simulink model "MEKFsim_v2"  (R2020b)
settings: Solver=FixedStepAuto  StartTime=0.0  StopTime=tsimulation  FixedStep=delta_t  RelTol=1e-3
values from neighbouring files (symbols this model uses):
  b_offset = sat.sensors.gyro_bias    [MEKF_Monte_Carlo_simulation.m]    (also in UKF_Monte_Carlo_simulation.m; main_SDA.m; main_SDA_v2.m)
  b_offset2 = -1e-2    (= -0.01)    [MEKF_Monte_Carlo_simulation.m]    (also in UKF_Monte_Carlo_simulation.m; main_SDA.m = 0; main_SDA_v2.m = 0)
  date_IGRF = [date.year,date.month,date.day]    [MEKF_Monte_Carlo_simulation.m]    (also in UKF_Monte_Carlo_simulation.m; main_SDA.m; main_SDA_v2.m)
  m = 12    [MEKF_Monte_Carlo_simulation.m]    (also in UKF_Monte_Carlo_simulation.m; main_SDA.m; main_SDA_v2.m)
  MODE = 2    [MEKF_Monte_Carlo_simulation.m]    (also in UKF_Monte_Carlo_simulation.m; main_SDA.m; main_SDA_v2.m)
  nmax_KF = 2    [MEKF_Monte_Carlo_simulation.m]    (also in UKF_Monte_Carlo_simulation.m; main_SDA.m; main_SDA_v2.m)
  PSDbias = sat.sensors.gyro_bias^2*Ts    [MEKF_Monte_Carlo_simulation.m]    (also in UKF_Monte_Carlo_simulation.m; main_SDA.m; main_SDA_v2.m)
  PSDcss = sat.sensors.sun_coarse_sigma^2*Tss    [MEKF_Monte_Carlo_simulation.m]    (also in UKF_Monte_Carlo_simulation.m; main_SDA.m; main_SDA_v2.m)
  PSDfss = sat.sensors.sun_sigma^2*Tss    [MEKF_Monte_Carlo_simulation.m]    (also in UKF_Monte_Carlo_simulation.m; main_SDA.m; main_SDA_v2.m)
  PSDgyro = sat.sensors.gyro_sigma^2*Ts    [MEKF_Monte_Carlo_simulation.m]    (also in UKF_Monte_Carlo_simulation.m; main_SDA.m; main_SDA_v2.m)
  PSDmtm = sat.sensors.mag_sigma^2*Tss    [MEKF_Monte_Carlo_simulation.m]    (also in UKF_Monte_Carlo_simulation.m; main_SDA.m; main_SDA_v2.m)
  Ts = 1    [MEKF_Monte_Carlo_simulation.m]    (also in UKF_Monte_Carlo_simulation.m; main_SDA.m = 0.5; main_SDA_v2.m = 0.5)
  Tss = 1    [MEKF_Monte_Carlo_simulation.m]    (also in UKF_Monte_Carlo_simulation.m; main_SDA.m = 0.5; main_SDA_v2.m = 0.5)
  Use_IGRF = 0    [MEKF_Monte_Carlo_simulation.m]    (also in UKF_Monte_Carlo_simulation.m; main_SDA.m; main_SDA_v2.m)
  Use_IGRF_KF = 0    [MEKF_Monte_Carlo_simulation.m]    (also in UKF_Monte_Carlo_simulation.m; main_SDA.m; main_SDA_v2.m)
undefined symbols (not defined in the file or in its folder): date, deg, DipoleMod, km, orbit, rad, s
libraries: aerolibconvert2 x14, aerolibutil x14, sharedtransform x9, dspmathops x8, vrlib x7, simulink x6, aerolibobsolete x2, aerolibcelestial x2, aerolibgravity2 x1, sharedutil x1, DipoleModel x1
(part 1 of 2)
settings Model: Creator=Ricardo  LastModifiedBy=colpari

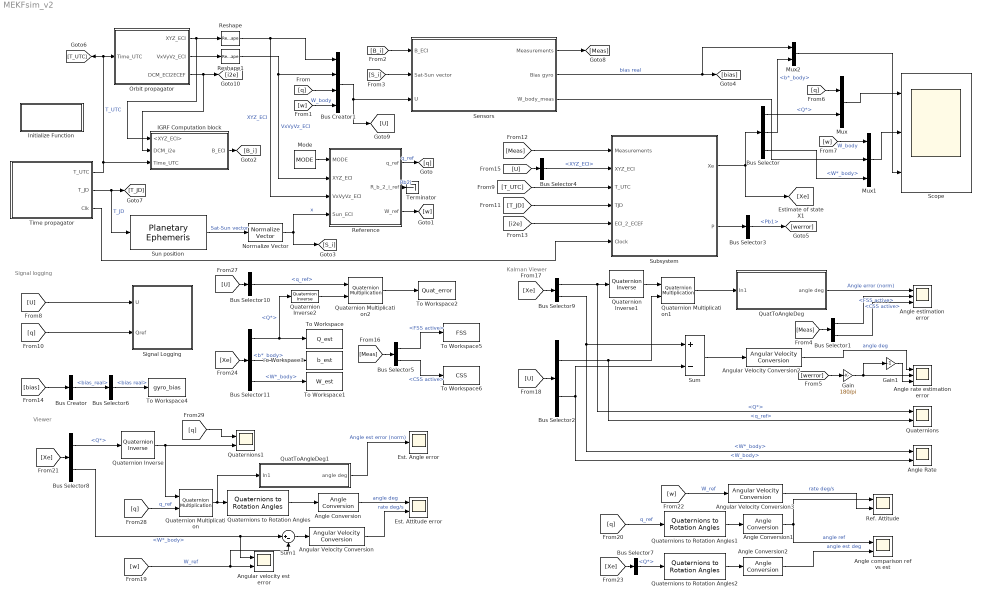
== system MEKFsim_v2 ==
  note: Signal logging
  note: Kalman Viewer
  note: Viewer
  Angle comparison ref vs est : Scope  NumInputPorts=2
  Angle Conversion : aerolibconvert2/Angle Conversion  IU=rad  OU=deg
  Angle Conversion1 : aerolibconvert2/Angle Conversion  IU=rad  OU=deg
  Angle Conversion2 : aerolibconvert2/Angle Conversion  IU=rad  OU=deg
  Angle Rate : Scope  NumInputPorts=2
  Angle estimation error : Scope  NumInputPorts=3
  Angle rate estimation error : Scope  NumInputPorts=3
  Angular Velocity Conversion : aerolibconvert2/Angular Velocity Conversion  IU=rad/s  OU=deg/s
  Angular Velocity Conversion2 : aerolibconvert2/Angular Velocity Conversion  IU=rad/s  OU=deg/s
  Angular Velocity Conversion3 : aerolibconvert2/Angular Velocity Conversion  IU=rad/s  OU=deg/s
  Angular velocity est error : Scope  NumInputPorts=2
  Bus Creator : BusCreator  Inputs=1
  Bus Creator1 : BusCreator  Inputs=4
  Bus Selector : BusSelector  OutputSignals=Q*,b*_body,W*_body
  Bus Selector1 : BusSelector  OutputSignals=FSS active,CSS active
  Bus Selector10 : BusSelector  OutputSignals=q_ref
  Bus Selector11 : BusSelector  OutputSignals=Q*,b*_body,W*_body
  Bus Selector2 : BusSelector  OutputSignals=q_ref,W_body
  Bus Selector3 : BusSelector  OutputSignals=Pb1
  Bus Selector4 : BusSelector  OutputSignals=XYZ_ECI
  Bus Selector5 : BusSelector  OutputSignals=FSS active,CSS active
  Bus Selector6 : BusSelector  OutputSignals=bias real
  Bus Selector7 : BusSelector  OutputSignals=Q*
  Bus Selector8 : BusSelector  OutputSignals=Q*,W*_body
  Bus Selector9 : BusSelector  OutputSignals=Q*,W*_body
  Est. Angle error : Scope
  Est. Attitude error : Scope  NumInputPorts=2
  Gain : Gain  Gain=180/pi
  Gain1 : Gain  Gain=-1
  IGRF Computation block : Subsystem
  Initialize Function : Subsystem  TreatAsAtomicUnit=on
  Mode : Constant  Value=MODE  OutDataTypeStr=int8
  Mux : Mux  Inputs=2
  Mux1 : Mux  Inputs=3
  Mux2 : Mux  Inputs=2
  Normalize Vector : vrlib/Utilities/Normalize Vector  maxzero=0
  Orbit propagator : Subsystem
  QuatToAngleDeg : Subsystem
  QuatToAngleDeg1 : Subsystem
  Quaternion Inverse : aerolibutil/Quaternion Inverse
  Quaternion Inverse1 : aerolibutil/Quaternion Inverse
  Quaternion Inverse2 : aerolibutil/Quaternion Inverse
  Quaternion Multiplication : aerolibutil/Quaternion Multiplication
  Quaternion Multiplication1 : aerolibutil/Quaternion Multiplication
  Quaternion Multiplication2 : aerolibutil/Quaternion Multiplication
  Quaternions : Scope  NumInputPorts=2
  Quaternions to Rotation Angles : sharedtransform/Quaternions to Rotation Angles  rotationOrder=ZYX  aMode=aMode
      settings: SourceProductBaseCode=AE,PW,MT,UV,VE,VP
  Quaternions to Rotation Angles1 : sharedtransform/Quaternions to Rotation Angles  rotationOrder=ZYX  aMode=aMode
      settings: SourceProductBaseCode=AE,PW,MT,UV,VE,VP
  Quaternions to Rotation Angles2 : sharedtransform/Quaternions to Rotation Angles  rotationOrder=ZYX  aMode=aMode
      settings: SourceProductBaseCode=AE,PW,MT,UV,VE,VP
  Quaternions1 : Scope  NumInputPorts=2
  Ref. Attitude : Scope  NumInputPorts=2
  Reference : Subsystem  TreatAsAtomicUnit=on
  Reshape : Reshape
  Reshape1 : Reshape
  Scope : Scope  NumInputPorts=3
  Sensors : Subsystem
  Signal Logging : Subsystem
  Subsystem : Subsystem
  Sum : Sum  Inputs=+-
  Sum1 : Sum  Inputs=|+-
  Sun position : aerolibcelestial/Planetary Ephemeris  kmflag=km,km/s  epochflag=Julian date  de=DE405  nCenter=Earth  nTarget=Sun  errorflag=Error  velflag=off
      settings: SourceProductBaseCode=AE
  Terminator : Terminator
  Time propagator : Subsystem
  To Workspace : ToWorkspace  VariableName=Q_est  SaveFormat=Timeseries  SampleTime=-1
  To Workspace1 : ToWorkspace  VariableName=W_est  SaveFormat=Timeseries  SampleTime=-1
  To Workspace2 : ToWorkspace  VariableName=Quat_error  SaveFormat=Timeseries  SampleTime=-1
  To Workspace3 : ToWorkspace  VariableName=b_est  SaveFormat=Timeseries  SampleTime=-1
  To Workspace4 : ToWorkspace  VariableName=gyro_bias  SaveFormat=Timeseries  SampleTime=-1
      settings: Save2DSignal=2-D array (concatenate along first dimension)
  To Workspace5 : ToWorkspace  VariableName=FSS  SaveFormat=Timeseries  SampleTime=-1
  To Workspace6 : ToWorkspace  VariableName=CSS  SaveFormat=Timeseries  SampleTime=-1
  wires:
  Orbit propagator/2(VxVyVz_ECI) -> Reshape1/1
  Orbit propagator/1(XYZ_ECI) -> IGRF Computation block/1(<XYZ_ECI>), Reshape/1
  Normalize Vector/1 -> Reference/4(Sun_ECI), [S_i]  "x"
  Sun position/1 -> Normalize Vector/1  "Sat-Sun vector"
  Time propagator/1(T_UTC) -> IGRF Computation block/3("Time_UTC "), [T_UTC], Orbit propagator/1("Time_UTC ")  "T_UTC"
  Time propagator/2(T_JD) -> Sun position/1, [T_JD]  "T_JD"
  Orbit propagator/3(DCM_ECI2ECEF) -> IGRF Computation block/2("DCM_i2e "), [i2e]
  IGRF Computation block/1(B_ECI) -> [B_i]
  [q] -> Bus Creator1/3
  [w] -> Bus Creator1/4  "W_body"
  Bus Creator1/1 -> [U], Sensors/3(U)
  [B_i] -> Sensors/1(B_ECI)
  [S_i] -> Sensors/2(Sat-Sun vector)
  [q] -> Mux/1
  Bus Selector/1 -> Mux/2  "<Q*>"
  Bus Selector/3 -> Mux1/3  "<W*_body>"
  [w] -> Mux1/1  "W_body"
  Sensors/3(W_body_meas) -> Mux1/2
  Mux/1 -> Scope/1
  Mux1/1 -> Scope/2
  Bus Selector11/1 -> Quaternion Inverse2/1, To Workspace/1  "<Q*>"
  Bus Selector10/1 -> Quaternion Multiplication2/1  "<q_ref>"
  [q] -> Signal Logging/2(Qref)
  Quaternion Inverse2/1 -> Quaternion Multiplication2/2
  Quaternion Multiplication2/1 -> To Workspace2/1
  [U] -> Bus Selector10/1
  [Xe] -> Bus Selector11/1
  [U] -> Signal Logging/1(U)
  Bus Selector11/3 -> To Workspace1/1  "<W*_body>"
  Quaternion Multiplication1/1 -> QuatToAngleDeg/1(In1)
  Bus Selector1/2 -> Angle estimation error/3  "<CSS active>"
  QuatToAngleDeg/1(angle deg) -> Angle estimation error/1  "Angle error (norm)"
  Angular Velocity Conversion2/1 -> Angle rate estimation error/1  "angle deg"
  Bus Selector2/1 -> Quaternions/2, Quaternion Multiplication1/2  "<q_ref>"
  Bus Selector1/1 -> Angle estimation error/2  "<FSS active>"
  Bus Selector2/2 -> Sum/2, Angle Rate/2  "<W_body>"
  Sum/1 -> Angular Velocity Conversion2/1
  [Xe] -> Bus Selector9/1
  Bus Selector9/1 -> Quaternions/1, Quaternion Inverse1/1  "<Q*>"
  Bus Selector9/2 -> Angle Rate/1, Sum/1  "<W*_body>"
  Quaternion Inverse1/1 -> Quaternion Multiplication1/1
  [U] -> Bus Selector2/1
  [T_UTC] -> Subsystem/3(T_UTC)
  [T_JD] -> Subsystem/4(TJD)
  Bus Selector4/1 -> Subsystem/2(XYZ_ECI)  "<XYZ_ECI>"
  [U] -> Bus Selector4/1
  Subsystem/1(Xe) -> [Xe], Bus Selector/1
  Subsystem/2(P) -> Bus Selector3/1
  Gain1/1 -> Angle rate estimation error/3
  Bus Selector3/1 -> [werror]  "<Pb1>"
  [werror] -> Gain/1
  Gain/1 -> Gain1/1, Angle rate estimation error/2
  Reshape1/1 -> Reference/2(XYZ_ECI), Bus Creator1/2  "VxVyVz_ECI"
  Reshape/1 -> Reference/3(VxVyVz_ECI), Bus Creator1/1  "XYZ_ECI"
  [i2e] -> Subsystem/5(ECI_2_ECEF)
  Time propagator/3(Clk) -> Subsystem/6(Clock)
  Sensors/2(Bias gyro) -> [bias], Mux2/1  "bias real"
  Bus Selector/2 -> Mux2/2  "<b*_body>"
  Mux2/1 -> Scope/3
  Sensors/1(Measurements) -> [Meas]
  [Meas] -> Subsystem/1(Measurements)
  [Meas] -> Bus Selector1/1
  Bus Selector11/2 -> To Workspace3/1  "<b*_body>"
  [bias] -> Bus Creator/1
  Bus Selector5/1 -> To Workspace5/1  "<FSS active>"
  [Meas] -> Bus Selector5/1
  Bus Selector5/2 -> To Workspace6/1  "<CSS active>"
  Bus Creator/1 -> Bus Selector6/1  "<bias_real>"
  Bus Selector6/1 -> To Workspace4/1  "<bias real>"
  Reference/2(R_b_2_i_ref) -> Terminator/1  "Rb2i"
  Reference/1(q_ref) -> [q]  "q_ref"
  Reference/3(W_ref) -> [w]
  Mode/1 -> Reference/1(MODE)
  Bus Selector8/1 -> Quaternion Inverse/1  "<Q*>"
  [q] -> Quaternion Multiplication/2  "q_ref"
  Quaternions to Rotation Angles/1 -> Angle Conversion/1
  [w] -> Sum1/2, Angular velocity est error/2  "W_ref"
  Quaternion Inverse/1 -> Quaternion Multiplication/1, Quaternions1/2
  [Xe] -> Bus Selector8/1
  Angle Conversion/1 -> Est. Attitude error/1  "angle deg"
  QuatToAngleDeg1/1(angle deg) -> Est. Angle error/1  "Angle est error (norm)"
  Quaternion Multiplication/1 -> QuatToAngleDeg1/1(In1), Quaternions to Rotation Angles/1
  Sum1/1 -> Angular Velocity Conversion/1
  Angular Velocity Conversion/1 -> Est. Attitude error/2  "rate deg/s"
  [q] -> Quaternions1/1
  Bus Selector8/2 -> Sum1/1, Angular velocity est error/1  "<W*_body>"
  [w] -> Angular Velocity Conversion3/1  "W_ref"
  [Xe] -> Bus Selector7/1
  Angular Velocity Conversion3/1 -> Ref. Attitude/2  "rate deg/s"
  Angle Conversion2/1 -> Angle comparison ref vs est/2  "angle est deg"
  Bus Selector7/1 -> Quaternions to Rotation Angles2/1  "<Q*>"
  Quaternions to Rotation Angles1/1 -> Angle Conversion1/1
  Angle Conversion1/1 -> Ref. Attitude/1, Angle comparison ref vs est/1  "angle ref"
  Quaternions to Rotation Angles2/1 -> Angle Conversion2/1
  [q] -> Quaternions to Rotation Angles1/1  "q_ref"

== system MEKFsim_v2/IGRF Computation block ==
  <XYZ_ECI> : Inport
  "DCM_i2e " : Inport  Port=2
  "Time_UTC " : Inport  Port=3
  Bus Creator : BusCreator  Inputs=5
  Demux : Demux  Outputs=2
  ECI To LLA : MATLAB Function  TreatAsAtomicUnit=on
  Obtain B_ECI : Subsystem
  Product : Product  Multiplication=Matrix(*)
  Reshape : Reshape  OutputDimensionality=Row vector (2-D)
  Terminator : Terminator
  B_ECI : Outport  VectorParamsAs1DForOutWhenUnconnected=off
  wires:
  ECI To LLA/3(long) -> Bus Creator/3
  ECI To LLA/2(lat) -> Bus Creator/2
  ECI To LLA/1(h) -> Bus Creator/1
  Demux/1 -> Bus Creator/4  "time_UTC"
  Demux/2 -> Terminator/1
  "DCM_i2e "/1 -> Product/2, Bus Creator/5  "DCM_i2e"
  Reshape/1 -> Product/1
  Product/1 -> ECI To LLA/1(X_ECEF)
  Bus Creator/1 -> Obtain B_ECI/1(In1)
  Obtain B_ECI/1(Out1) -> B_ECI/1
  "Time_UTC "/1 -> Demux/1
  <XYZ_ECI>/1 -> Reshape/1

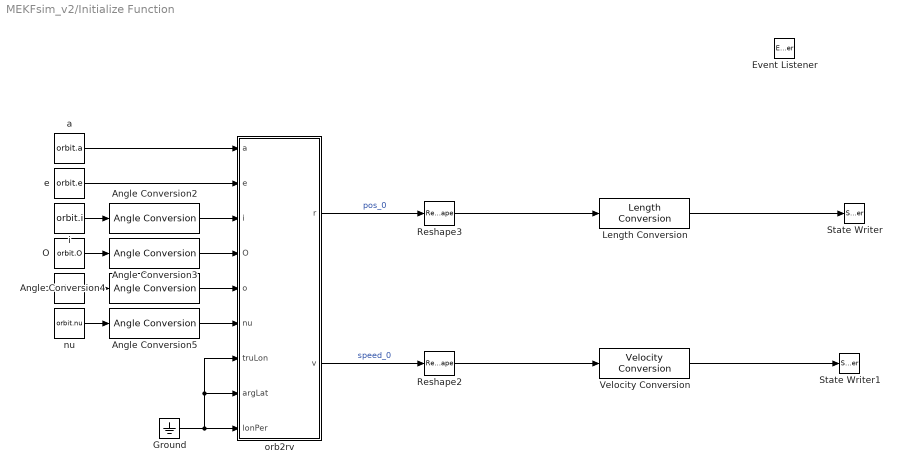
== system MEKFsim_v2/Initialize Function ==
  Angle Conversion{2..5} (4 alike) : aerolibconvert2/Angle Conversion  IU=deg  OU=rad
  Event Listener : EventListener  DisableCoverage=on  EventName=reset
  Ground : Ground
  Length Conversion : aerolibconvert2/Length Conversion  IU=km  OU=m
  O : Constant  Value=orbit.O
  Reshape2 : Reshape  OutputDimensionality=Column vector (2-D)
  Reshape3 : Reshape  OutputDimensionality=Column vector (2-D)
  State Writer : StateWriter  StateOwnerBlock=../../Orbit propagator/Integrator_pos
  State Writer1 : StateWriter  StateOwnerBlock=../../Orbit propagator/Integrator_speed
  Velocity Conversion : aerolibconvert2/Velocity Conversion  IU=km/s  OU=m/s
  a : Constant  Value=orbit.a
  e : Constant  Value=orbit.e
  i : Constant  Value=orbit.i
  nu : Constant  Value=orbit.nu
  o : Constant  Value=orbit.o
  orb2rv : MATLAB Function  TreatAsAtomicUnit=on
  wires:
  Angle Conversion2/1 -> orb2rv/3(i)
  Length Conversion/1 -> State Writer/1
  Angle Conversion4/1 -> orb2rv/5(o)
  nu/1 -> Angle Conversion5/1
  Angle Conversion3/1 -> orb2rv/4(O)
  e/1 -> orb2rv/2(e)
  Reshape3/1 -> Length Conversion/1
  O/1 -> Angle Conversion3/1
  a/1 -> orb2rv/1(a)
  i/1 -> Angle Conversion2/1
  orb2rv/1(r) -> Reshape3/1  "pos_0"
  o/1 -> Angle Conversion4/1
  Angle Conversion5/1 -> orb2rv/6(nu)
  Velocity Conversion/1 -> State Writer1/1
  Reshape2/1 -> Velocity Conversion/1
  orb2rv/2(v) -> Reshape2/1  "speed_0"
  Ground/1 -> orb2rv/8(argLat), orb2rv/7(truLon), orb2rv/9(lonPer)

== system MEKFsim_v2/Orbit propagator ==
  "Time_UTC " : Inport
  1/m : Gain  Gain=1/m
  Integrator_pos : Integrator
  Integrator_speed : Integrator
  Reshape : Reshape  OutputDimensionality=Column vector (2-D)
  Reshape2 : Reshape  OutputDimensionality=Column vector (2-D)
  Spherical Harmonic Gravity : Subsystem  TreatAsAtomicUnit=on  SystemSampleTime=1
  m : Gain  Gain=m
  XYZ_ECI : Outport  VectorParamsAs1DForOutWhenUnconnected=off
  VxVyVz_ECI : Outport  Port=2
  DCM_ECI2ECEF : Outport  Port=3
  wires:
  Integrator_pos/1 -> Reshape2/1, XYZ_ECI/1  "XYZ_ECI"
  Integrator_speed/1 -> VxVyVz_ECI/1, Integrator_pos/1  "VxVyVz_ECI"
  1/m/1 -> Integrator_speed/1  "AxAyAz_ECI"
  Reshape/1 -> 1/m/1
  m/1 -> Reshape/1  "Force_ECI"
  Spherical Harmonic Gravity/1(g_ECI (m/s²)) -> m/1
  "Time_UTC "/1 -> Spherical Harmonic Gravity/2(Time_UTC)
  Reshape2/1 -> Spherical Harmonic Gravity/1(XYZ_ECI)
  Spherical Harmonic Gravity/2(DCM_ECI2ECEF) -> DCM_ECI2ECEF/1

== system MEKFsim_v2/QuatToAngleDeg ==
  In1 : Inport
  Abs : Abs
  Abs1 : Abs
  Acos : Trigonometry  Operator=acos
  Angle Conversion1 : aerolibconvert2/Angle Conversion  IU=rad  OU=deg
  Demux1 : Demux
  Gain : Gain  Gain=2
  Scope : Scope
  Terminator1 : Terminator
  Terminator2 : Terminator
  Terminator3 : Terminator
  angle deg : Outport  VectorParamsAs1DForOutWhenUnconnected=off
  wires:
  Acos/1 -> Gain/1
  Demux1/4 -> Terminator1/1
  In1/1 -> Demux1/1
  Angle Conversion1/1 -> Abs/1  "angle deg"
  Demux1/2 -> Terminator2/1
  Demux1/3 -> Terminator3/1
  Abs/1 -> angle deg/1
  Demux1/1 -> Abs1/1, Scope/1
  Gain/1 -> Angle Conversion1/1
  Abs1/1 -> Acos/1

== system MEKFsim_v2/QuatToAngleDeg1 ==
  In1 : Inport
  Abs : Abs
  Angle Conversion1 : aerolibconvert2/Angle Conversion  IU=rad  OU=deg
  Demux1 : Demux
  Quaternion to axis and angle conversion : MATLABFcn  MATLABFcn=quat2axisangle
  Terminator1 : Terminator
  Terminator2 : Terminator
  Terminator3 : Terminator
  angle deg : Outport  VectorParamsAs1DForOutWhenUnconnected=off
  wires:
  Demux1/2 -> Terminator2/1
  Demux1/4 -> Angle Conversion1/1
  In1/1 -> Quaternion to axis and angle conversion/1
  Demux1/1 -> Terminator1/1
  Demux1/3 -> Terminator3/1
  Quaternion to axis and angle conversion/1 -> Demux1/1
  Abs/1 -> angle deg/1
  Angle Conversion1/1 -> Abs/1  "angle deg"

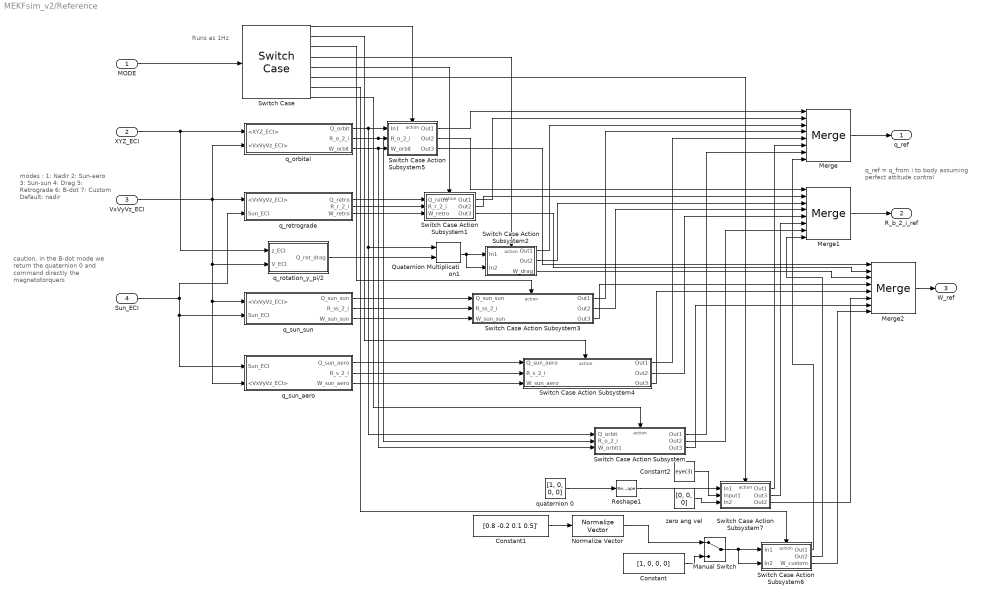
== system MEKFsim_v2/Reference ==
  note: caution, in the B-dot mode we return the quaternion 0 and command directly the magnetotorquers
  note: modes :
      | 1: Nadir
      | 2: Sun-aero
      | 3: Sun-sun
      | 4: Drag
      | 5: Retrograde
      | 6: B-dot
      | 7: Custom
      | Default: nadir
  note: Runs as 1Hz
  note: q_ref  = q_from i to body
      | assuming perfect attitude control
  MODE : Inport  OutMin=1  OutMax=100  OutDataTypeStr=int8
  XYZ_ECI : Inport  Port=2
  VxVyVz_ECI : Inport  Port=3
  Sun_ECI : Inport  Port=4
  Constant : Constant  Value=[1, 0, 0, 0]
  Constant1 : Constant  Value=[0.8 -0.2 0.1 0.5]'
  Constant2 : Constant  Value=eye(3)
  Manual Switch : ManualSwitch
  Merge : Merge  Inputs=8
  Merge1 : Merge  Inputs=8
  Merge2 : Merge  Inputs=8
  Normalize Vector : vrlib/Utilities/Normalize Vector  maxzero=0
  Quaternion Multiplication1 : aerolibutil/Quaternion Multiplication
  Reshape1 : Reshape  OutputDimensionality=Column vector (2-D)
  Switch Case : SwitchCase  CaseConditions={1, 2, 3, 4, 5, 6, 7}
  Switch Case Action Subsystem : Subsystem  TreatAsAtomicUnit=on
  Switch Case Action Subsystem1 : Subsystem  TreatAsAtomicUnit=on
  Switch Case Action Subsystem2 : Subsystem  TreatAsAtomicUnit=on
  Switch Case Action Subsystem3 : Subsystem  TreatAsAtomicUnit=on
  Switch Case Action Subsystem4 : Subsystem  TreatAsAtomicUnit=on
  Switch Case Action Subsystem5 : Subsystem  TreatAsAtomicUnit=on
  Switch Case Action Subsystem6 : Subsystem  TreatAsAtomicUnit=on
  Switch Case Action Subsystem7 : Subsystem  TreatAsAtomicUnit=on
  q_orbital : Subsystem
  q_retrograde : Subsystem
  q_rotation_y_pi/2 : Subsystem
  q_sun_aero : Subsystem
  q_sun_sun : Subsystem
  quaternion 0 : Constant  Value=[1, 0, 0, 0]
  zero ang vel : Constant  Value=[0, 0, 0]
  q_ref : Outport  VectorParamsAs1DForOutWhenUnconnected=off
  R_b_2_i_ref : Outport  Port=2
  W_ref : Outport  Port=3
  wires:
  q_sun_sun/1(Q_sun_sun) -> Switch Case Action Subsystem3/1(Q_sun_sun)
  Sun_ECI/1 -> q_retrograde/2(Sun_ECI), q_sun_aero/1(Sun_ECI), q_sun_sun/2(Sun_ECI)
  MODE/1 -> Switch Case/1
  q_rotation_y_pi/2/1(Q_rot_drag) -> Quaternion Multiplication1/2
  Switch Case/3 -> Switch Case Action Subsystem3/Action
  q_sun_aero/1(Q_sun_aero) -> Switch Case Action Subsystem4/1(Q_sun_aero)
  Merge/1 -> q_ref/1
  XYZ_ECI/1 -> q_orbital/1(<XYZ_ECI>), q_rotation_y_pi/2/1(z_ECI)
  Switch Case/5 -> Switch Case Action Subsystem1/Action
  Switch Case/4 -> Switch Case Action Subsystem2/Action
  quaternion 0/1 -> Reshape1/1
  VxVyVz_ECI/1 -> q_orbital/2(<VxVyVz_ECI>), q_retrograde/1(<VxVyVz_ECI>), q_sun_aero/2(<VxVyVz_ECI>), q_sun_sun/1(<VxVyVz_ECI>), q_rotation_y_pi/2/2(V_ECI)
  Switch Case/2 -> Switch Case Action Subsystem4/Action
  Quaternion Multiplication1/1 -> Switch Case Action Subsystem2/2(In2), Switch Case Action Subsystem2/1(In1)
  q_orbital/1(Q_orbit) -> Quaternion Multiplication1/1, Switch Case Action Subsystem/1(Q_orbit), Switch Case Action Subsystem5/1(In1)
  Switch Case/6 -> Switch Case Action Subsystem7/Action
  q_retrograde/1(Q_retro) -> Switch Case Action Subsystem1/1(Q_retro)
  Reshape1/1 -> Switch Case Action Subsystem7/1(In1)
  Merge1/1 -> R_b_2_i_ref/1
  Switch Case Action Subsystem5/1(Out1) -> Merge/1
  Switch Case Action Subsystem5/2(Out2) -> Merge1/1
  Switch Case Action Subsystem1/1(Out1) -> Merge/2
  Switch Case Action Subsystem1/2(Out2) -> Merge1/2
  Switch Case Action Subsystem2/1(Out1) -> Merge/3
  Switch Case Action Subsystem2/2(Out2) -> Merge1/3
  Switch Case Action Subsystem3/1(Out1) -> Merge/4
  Switch Case Action Subsystem3/2(Out2) -> Merge1/4
  Switch Case Action Subsystem4/1(Out1) -> Merge/5
  Switch Case Action Subsystem4/2(Out2) -> Merge1/5
  Switch Case Action Subsystem/1(Out1) -> Merge/7
  Switch Case Action Subsystem/2(Out2) -> Merge1/7
  Switch Case Action Subsystem7/1(Out1) -> Merge/6
  Switch Case Action Subsystem7/2(Out3) -> Merge1/6
  Switch Case/1 -> Switch Case Action Subsystem5/Action
  Switch Case/8 -> Switch Case Action Subsystem/Action
  Switch Case/7 -> Switch Case Action Subsystem6/Action
  Constant/1 -> Manual Switch/2
  Switch Case Action Subsystem6/1(Out1) -> Merge/8
  Switch Case Action Subsystem6/2(Out2) -> Merge1/8
  Constant1/1 -> Normalize Vector/1
  Normalize Vector/1 -> Manual Switch/1
  Manual Switch/1 -> Switch Case Action Subsystem6/2(In2), Switch Case Action Subsystem6/1(In1)
  q_orbital/2(R_o_2_i) -> Switch Case Action Subsystem/2(R_o_2_i), Switch Case Action Subsystem5/2(R_o_2_i)
  q_sun_aero/2(R_s_2_i) -> Switch Case Action Subsystem4/2(R_s_2_i)
  q_sun_sun/2(R_ss_2_i) -> Switch Case Action Subsystem3/2(R_ss_2_i)
  q_retrograde/2(R_r_2_i) -> Switch Case Action Subsystem1/2(R_r_2_i)
  Constant2/1 -> Switch Case Action Subsystem7/2(Input1)
  q_orbital/3(W_orbit) -> Switch Case Action Subsystem/3(W_orbit1), Switch Case Action Subsystem5/3(W_orbit)
  q_retrograde/3(W_retro) -> Switch Case Action Subsystem1/3(W_retro)
  q_sun_aero/3(W_sun_aero) -> Switch Case Action Subsystem4/3(W_sun_aero)
  q_sun_sun/3(W_sun_sun) -> Switch Case Action Subsystem3/3(W_sun_sun)
  Merge2/1 -> W_ref/1
  Switch Case Action Subsystem5/3(Out3) -> Merge2/1
  Switch Case Action Subsystem4/3(Out3) -> Merge2/5
  Switch Case Action Subsystem3/3(Out3) -> Merge2/4
  Switch Case Action Subsystem2/3(W_drag) -> Merge2/3
  Switch Case Action Subsystem1/3(Out3) -> Merge2/2
  zero ang vel/1 -> Switch Case Action Subsystem7/3(In2)
  Switch Case Action Subsystem7/3(Out2) -> Merge2/6
  Switch Case Action Subsystem/3(Out3) -> Merge2/7
  Switch Case Action Subsystem6/3(W_custom) -> Merge2/8

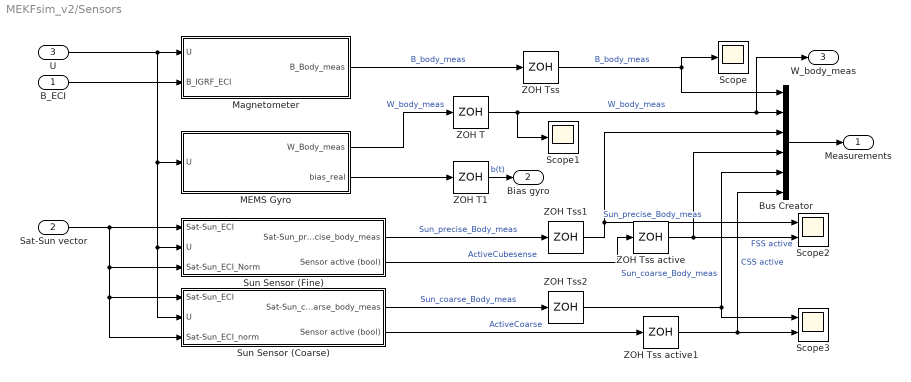
== system MEKFsim_v2/Sensors ==
  B_ECI : Inport
  Sat-Sun vector : Inport  Port=2
  U : Inport  Port=3
  Bus Creator : BusCreator  Inputs=6
  MEMS Gyro : Subsystem
  Magnetometer : Subsystem
  Scope : Scope
  Scope1 : Scope
  Scope2 : Scope  NumInputPorts=2
  Scope3 : Scope  NumInputPorts=2
  Sun Sensor (Coarse) : Subsystem
  Sun Sensor (Fine) : Subsystem
  ZOH T : ZeroOrderHold  SampleTime=Ts
  ZOH T1 : ZeroOrderHold  SampleTime=Ts
  ZOH Tss : ZeroOrderHold  SampleTime=Tss
  ZOH Tss active : ZeroOrderHold  SampleTime=Tss
  ZOH Tss active1 : ZeroOrderHold  SampleTime=Tss
  ZOH Tss1 : ZeroOrderHold  SampleTime=Tss
  ZOH Tss2 : ZeroOrderHold  SampleTime=Tss
  Measurements : Outport  VectorParamsAs1DForOutWhenUnconnected=off
  Bias gyro : Outport  Port=2
  W_body_meas : Outport  Port=3
  wires:
  Sat-Sun vector/1 -> Sun Sensor (Fine)/3(Sat-Sun_ECI_Norm), Sun Sensor (Coarse)/3(Sat-Sun_ECI_norm), Sun Sensor (Coarse)/1(Sat-Sun_ECI), Sun Sensor (Fine)/1(Sat-Sun_ECI)
  MEMS Gyro/1(W_Body_meas) -> ZOH T/1  "W_body_meas"
  U/1 -> MEMS Gyro/1(U), Sun Sensor (Coarse)/2(U), Sun Sensor (Fine)/2(U), Magnetometer/1(U)
  Magnetometer/1(B_Body_meas) -> ZOH Tss/1  "B_body_meas"
  Sun Sensor (Coarse)/1(Sat-Sun_coarse_body_meas) -> ZOH Tss2/1  "Sun_coarse_Body_meas"
  Sun Sensor (Fine)/2(Sensor active (bool)) -> ZOH Tss active/1  "ActiveCubesense"
  Sun Sensor (Coarse)/2(Sensor active (bool)) -> ZOH Tss active1/1  "ActiveCoarse"
  B_ECI/1 -> Magnetometer/2(B_IGRF_ECI)
  Sun Sensor (Fine)/1(Sat-Sun_precise_body_meas) -> ZOH Tss1/1  "Sun_precise_Body_meas"
  ZOH Tss/1 -> Bus Creator/1, Scope/1  "B_body_meas"
  ZOH T/1 -> Bus Creator/2, W_body_meas/1, Scope1/1  "W_body_meas"
  ZOH Tss1/1 -> Bus Creator/3, Scope2/1  "Sun_precise_Body_meas"
  ZOH Tss2/1 -> Bus Creator/5, Scope3/1  "Sun_coarse_Body_meas"
  MEMS Gyro/2(bias_real) -> ZOH T1/1
  ZOH T1/1 -> Bias gyro/1  "b(t)"
  ZOH Tss active1/1 -> Bus Creator/6, Scope3/2  "CSS active"
  ZOH Tss active/1 -> Bus Creator/4, Scope2/2  "FSS active"
  Bus Creator/1 -> Measurements/1

== system MEKFsim_v2/Signal Logging ==
  U : Inport
  Qref : Inport  Port=2
  Bus Selector4 : BusSelector  OutputSignals=XYZ_ECI,VxVyVz_ECI,q_ref,W_body
  Reshape1 : Reshape
  Reshape3 : Reshape
  To Workspace : ToWorkspace  VariableName=sat_pos  SaveFormat=Timeseries  SampleTime=1
      settings: Save2DSignal=2-D array (concatenate along first dimension)
  To Workspace1 : ToWorkspace  VariableName=sat_speed  SaveFormat=Timeseries  SampleTime=1
      settings: Save2DSignal=2-D array (concatenate along first dimension)
  To Workspace2 : ToWorkspace  VariableName=sat_Q  SaveFormat=Timeseries  SampleTime=-1
      settings: Save2DSignal=2-D array (concatenate along first dimension)
  To Workspace3 : ToWorkspace  VariableName=sat_omega  SaveFormat=Timeseries  SampleTime=-1
      settings: Save2DSignal=2-D array (concatenate along first dimension)
  To Workspace5 : ToWorkspace  VariableName=sat_Qref  SaveFormat=Timeseries  SampleTime=-1
      settings: Save2DSignal=2-D array (concatenate along first dimension)
  wires:
  Bus Selector4/3 -> To Workspace2/1  "<q_ref>"
  Bus Selector4/4 -> Reshape3/1  "<W_body>"
  U/1 -> Bus Selector4/1
  Bus Selector4/2 -> To Workspace1/1  "<VxVyVz_ECI>"
  Bus Selector4/1 -> To Workspace/1  "<XYZ_ECI>"
  Qref/1 -> Reshape1/1
  Reshape1/1 -> To Workspace5/1
  Reshape3/1 -> To Workspace3/1

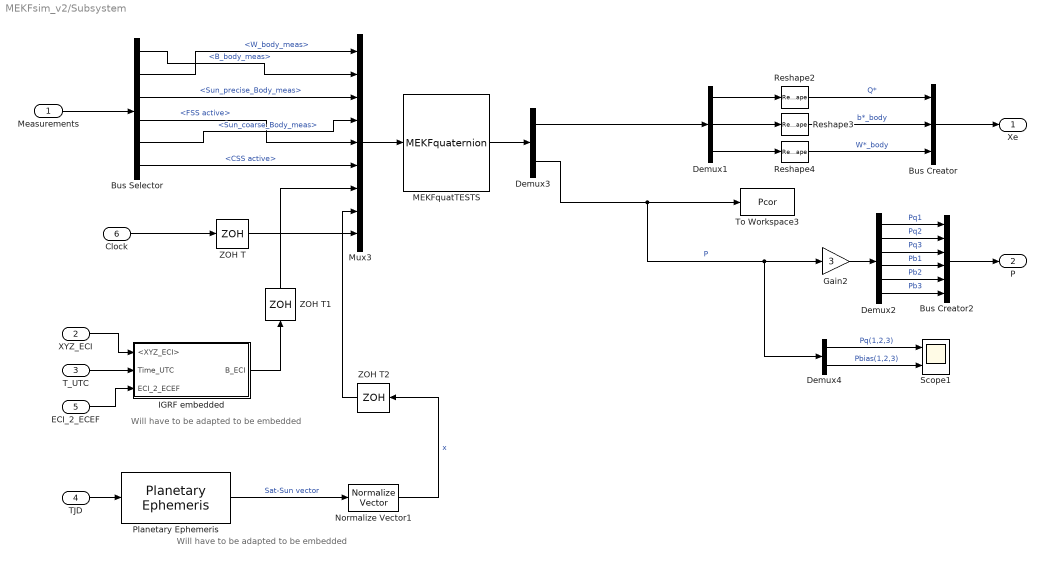
== system MEKFsim_v2/Subsystem ==
  note: Will have to be adapted to be embedded
  note: Will have to be adapted to be embedded
  Measurements : Inport
  XYZ_ECI : Inport  Port=2
  T_UTC : Inport  Port=3
  TJD : Inport  Port=4
  ECI_2_ECEF : Inport  Port=5
  Clock : Inport  Port=6
  Bus Creator : BusCreator  Inputs=3
  Bus Creator2 : BusCreator  Inputs=6
  Bus Selector : BusSelector  OutputSignals=B_body_meas,W_body_meas,Sun_precise_Body_meas,FSS active,Sun_coarse_Body_meas,CSS active
  Demux1 : Demux  Outputs=3
  Demux2 : Demux  Outputs=6
  Demux3 : Demux  Outputs=[10;6]
  Demux4 : Demux  Outputs=[3 3]
  Gain2 : Gain  Gain=3
  IGRF embedded : Subsystem
  MEKFquatTESTS : MATLABFcn  MATLABFcn=MEKFquaternion
  Mux3 : Mux  Inputs=9
  Normalize Vector1 : vrlib/Utilities/Normalize Vector  maxzero=0
  Planetary Ephemeris : aerolibcelestial/Planetary Ephemeris  kmflag=km,km/s  epochflag=Julian date  de=DE405  nCenter=Earth  nTarget=Sun  errorflag=Error  velflag=off
      settings: SourceProductBaseCode=AE
  Reshape2 : Reshape  OutputDimensionality=Customize  OutputDimensions=[4]
  Reshape3 : Reshape  OutputDimensionality=Customize  OutputDimensions=[3]
  Reshape4 : Reshape  OutputDimensionality=Customize  OutputDimensions=[3]
  Scope1 : Scope  NumInputPorts=2
  To Workspace3 : ToWorkspace  VariableName=Pcor  SaveFormat=Timeseries  SampleTime=-1
  ZOH T : ZeroOrderHold  SampleTime=Ts
  ZOH T1 : ZeroOrderHold  SampleTime=Ts
  ZOH T2 : ZeroOrderHold  SampleTime=Ts
  Xe : Outport  VectorParamsAs1DForOutWhenUnconnected=off
  P : Outport  Port=2
  wires:
  Demux2/1 -> Bus Creator2/1  "Pq1"
  Bus Selector/6 -> Mux3/6  "<CSS active>"
  ZOH T/1 -> Mux3/9
  Measurements/1 -> Bus Selector/1
  ZOH T2/1 -> Mux3/8
  Bus Selector/5 -> Mux3/4  "<Sun_coarse_Body_meas>"
  Reshape3/1 -> Bus Creator/2  "b*_body"
  Gain2/1 -> Demux2/1
  Clock/1 -> ZOH T/1
  Demux4/1 -> Scope1/1  "Pq(1,2,3)"
  Demux4/2 -> Scope1/2  "Pbias(1,2,3)"
  Reshape4/1 -> Bus Creator/3  "W*_body"
  Mux3/1 -> MEKFquatTESTS/1
  TJD/1 -> Planetary Ephemeris/1
  ECI_2_ECEF/1 -> IGRF embedded/3(ECI_2_ECEF)
  Bus Creator2/1 -> P/1
  Demux2/4 -> Bus Creator2/4  "Pb1"
  Demux2/2 -> Bus Creator2/2  "Pq2"
  T_UTC/1 -> IGRF embedded/2("Time_UTC ")
  Demux2/6 -> Bus Creator2/6  "Pb3"
  Demux1/3 -> Reshape4/1
  Demux2/5 -> Bus Creator2/5  "Pb2"
  XYZ_ECI/1 -> IGRF embedded/1(<XYZ_ECI>)
  Demux3/2 -> Demux4/1, Gain2/1, To Workspace3/1  "P"
  Reshape2/1 -> Bus Creator/1  "Q*"
  Normalize Vector1/1 -> ZOH T2/1  "x"
  MEKFquatTESTS/1 -> Demux3/1
  Demux1/2 -> Reshape3/1
  Bus Selector/4 -> Mux3/5  "<FSS active>"
  ZOH T1/1 -> Mux3/7
  IGRF embedded/1(B_ECI) -> ZOH T1/1
  Demux1/1 -> Reshape2/1
  Planetary Ephemeris/1 -> Normalize Vector1/1  "Sat-Sun vector"
  Demux3/1 -> Demux1/1
  Demux2/3 -> Bus Creator2/3  "Pq3"
  Bus Creator/1 -> Xe/1
  Bus Selector/2 -> Mux3/1  "<W_body_meas>"
  Bus Selector/1 -> Mux3/2  "<B_body_meas>"
  Bus Selector/3 -> Mux3/3  "<Sun_precise_Body_meas>"

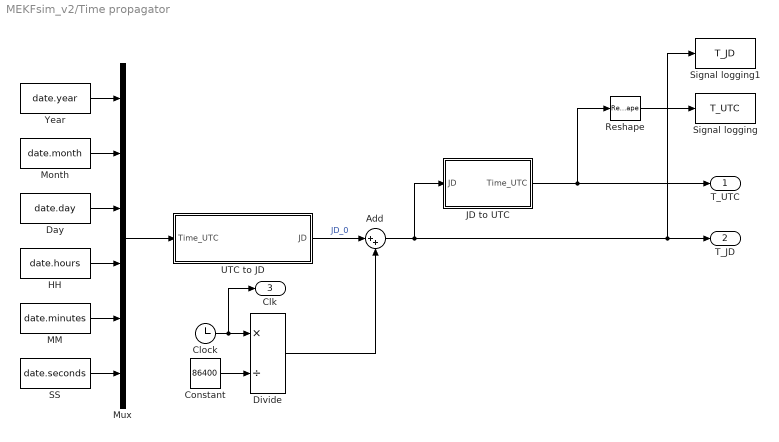
== system MEKFsim_v2/Time propagator ==
  Add : Sum  Inputs=|++
  Clock : Clock
  Constant : Constant  Value=86400
  Day : Constant  Value=date.day
  Divide : Product  Inputs=*/
  HH : Constant  Value=date.hours
  JD to UTC : MATLAB Function  TreatAsAtomicUnit=on
  MM : Constant  Value=date.minutes
  Month : Constant  Value=date.month
  Mux : Mux  Inputs=6
  Reshape : Reshape
  SS : Constant  Value=date.seconds
  Signal logging : ToWorkspace  VariableName=T_UTC  SaveFormat=Timeseries  SampleTime=1
      settings: Save2DSignal=2-D array (concatenate along first dimension)
  Signal logging1 : ToWorkspace  VariableName=T_JD  SaveFormat=Timeseries  SampleTime=1
      settings: Save2DSignal=2-D array (concatenate along first dimension)
  UTC to JD : MATLAB Function  TreatAsAtomicUnit=on
  Year : Constant  Value=date.year
  T_UTC : Outport  VectorParamsAs1DForOutWhenUnconnected=off
  T_JD : Outport  Port=2  VectorParamsAs1DForOutWhenUnconnected=off
  Clk : Outport  Port=3
  wires:
  UTC to JD/1(JD) -> Add/1  "JD_0"
  Clock/1 -> Clk/1, Divide/1
  Constant/1 -> Divide/2
  JD to UTC/1(Time_UTC) -> T_UTC/1, Reshape/1
  Divide/1 -> Add/2
  Mux/1 -> UTC to JD/1(Time_UTC)
  Day/1 -> Mux/3
  Month/1 -> Mux/2
  Year/1 -> Mux/1
  HH/1 -> Mux/4
  MM/1 -> Mux/5
  SS/1 -> Mux/6
  Reshape/1 -> Signal logging/1
  Add/1 -> Signal logging1/1, T_JD/1, JD to UTC/1(JD)

== system MEKFsim_v2/IGRF Computation block/Obtain B_ECI ==
  In1 : Inport
  Dipole Subsystem : Subsystem  TreatAsAtomicUnit=on
  IGRF Subsystem : Subsystem  TreatAsAtomicUnit=on
  If : If
  Merge : Merge
  Use_IGRF : Constant  Value=Use_IGRF
  Out1 : Outport  VectorParamsAs1DForOutWhenUnconnected=off
  wires:
  If/1 -> IGRF Subsystem/Action
  In1/1 -> Dipole Subsystem/1(In1), IGRF Subsystem/1(In1)
  IGRF Subsystem/1(Out1) -> Merge/1
  Use_IGRF/1 -> If/1
  Merge/1 -> Out1/1
  Dipole Subsystem/1("B_ECI ") -> Merge/2
  If/2 -> Dipole Subsystem/Action

== system MEKFsim_v2/Orbit propagator/Spherical Harmonic Gravity ==
  note: Slower subsytem because it's too slow
  XYZ_ECI : Inport
  Time_UTC : Inport  Port=2
  ECI_2_ECEF : MATLABFcn  MATLABFcn=eci2ecef  OutputDimensions=[3,3]  Output1D=off
  Product : Product  Multiplication=Matrix(*)
  Product1 : Product  Inputs=/*  Multiplication=Matrix(*)
  Spherical Harmonic Gravity Model : aerolibgravity2/Spherical Harmonic Gravity Model  units=Metric (MKS)  degree=100  action=Warning  ptype=EGM2008  datafile='aerogmm2b.mat'
      settings: SourceProductBaseCode=AE
  Transpose : Math  Operator=transpose  SignedPower=on  SaturateOnIntegerOverflow=on
  g_ECI (m/s²) : Outport
  DCM_ECI2ECEF : Outport  Port=2
  wires:
  ECI_2_ECEF/1 -> DCM_ECI2ECEF/1, Product1/1, Product/1
  Transpose/1 -> Product1/2
  Product/1 -> Spherical Harmonic Gravity Model/1
  Spherical Harmonic Gravity Model/1 -> Transpose/1
  XYZ_ECI/1 -> Product/2
  Product1/1 -> g_ECI (m/s²)/1
  Time_UTC/1 -> ECI_2_ECEF/1

== system MEKFsim_v2/Reference/Switch Case Action Subsystem ==
  Q_orbit : Inport
  R_o_2_i : Inport  Port=2
  W_orbit1 : Inport  Port=3
  Action Port : ActionPort  ActionPortLabel=default:
  Out1 : Outport  VectorParamsAs1DForOutWhenUnconnected=off
  Out2 : Outport  Port=2  VectorParamsAs1DForOutWhenUnconnected=off
  Out3 : Outport  Port=3  VectorParamsAs1DForOutWhenUnconnected=off
  wires:
  Q_orbit/1 -> Out1/1
  R_o_2_i/1 -> Out2/1
  W_orbit1/1 -> Out3/1

== system MEKFsim_v2/Reference/Switch Case Action Subsystem1 ==
  Q_retro : Inport
  R_r_2_i : Inport  Port=2
  W_retro : Inport  Port=3
  Action Port : ActionPort  ActionPortLabel=case [ 5 ]:
  Out1 : Outport  VectorParamsAs1DForOutWhenUnconnected=off
  Out2 : Outport  Port=2  VectorParamsAs1DForOutWhenUnconnected=off
  Out3 : Outport  Port=3  VectorParamsAs1DForOutWhenUnconnected=off
  wires:
  Q_retro/1 -> Out1/1
  R_r_2_i/1 -> Out2/1
  W_retro/1 -> Out3/1

== system MEKFsim_v2/Reference/Switch Case Action Subsystem2 ==
  note: q from I to O + rotation
  note: DCM from Inertial to Orbital
  note: DCM from Orbital to Inertial
  In1 : Inport
  In2 : Inport  Port=2
  Action Port : ActionPort  ActionPortLabel=case [ 4 ]:
  Derivative : Derivative
  Matrix Multiply : Product  Multiplication=Matrix(*)
  Quaternions to Direction Cosine Matrix : sharedtransform/Quaternions to  Direction Cosine Matrix  aMode=aMode
      settings: SourceProductBaseCode=AE,PW,MT,UV,VE,VP
  Transpose : Math  Operator=transpose  SaturateOnIntegerOverflow=on
  Transpose1 : Math  Operator=transpose  SaturateOnIntegerOverflow=on
  gets vector from Skew Matrix : MATLABFcn  MATLABFcn=vec_from_skew
  Out1 : Outport  VectorParamsAs1DForOutWhenUnconnected=off
  Out2 : Outport  Port=2  VectorParamsAs1DForOutWhenUnconnected=off
  W_drag : Outport  Port=3
  wires:
  In1/1 -> Out1/1
  In2/1 -> Quaternions to Direction Cosine Matrix/1
  Derivative/1 -> Matrix Multiply/1
  Transpose/1 -> Derivative/1
  gets vector from Skew Matrix/1 -> W_drag/1
  Matrix Multiply/1 -> gets vector from Skew Matrix/1
  Quaternions to Direction Cosine Matrix/1 -> Transpose1/1
  Transpose1/1 -> Out2/1, Transpose/1, Matrix Multiply/2

== system MEKFsim_v2/Reference/Switch Case Action Subsystem3 ==
  Q_sun_sun : Inport
  R_ss_2_i : Inport  Port=2
  W_sun_sun : Inport  Port=3
  Action Port : ActionPort  ActionPortLabel=case [ 3 ]:
  Out1 : Outport  VectorParamsAs1DForOutWhenUnconnected=off
  Out2 : Outport  Port=2  VectorParamsAs1DForOutWhenUnconnected=off
  Out3 : Outport  Port=3  VectorParamsAs1DForOutWhenUnconnected=off
  wires:
  Q_sun_sun/1 -> Out1/1
  R_ss_2_i/1 -> Out2/1
  W_sun_sun/1 -> Out3/1

== system MEKFsim_v2/Reference/Switch Case Action Subsystem4 ==
  Q_sun_aero : Inport
  R_s_2_i : Inport  Port=2
  W_sun_aero : Inport  Port=3
  Action Port : ActionPort  ActionPortLabel=case [ 2 ]:
  Out1 : Outport  VectorParamsAs1DForOutWhenUnconnected=off
  Out2 : Outport  Port=2  VectorParamsAs1DForOutWhenUnconnected=off
  Out3 : Outport  Port=3  VectorParamsAs1DForOutWhenUnconnected=off
  wires:
  Q_sun_aero/1 -> Out1/1
  R_s_2_i/1 -> Out2/1
  W_sun_aero/1 -> Out3/1

== system MEKFsim_v2/Reference/Switch Case Action Subsystem5 ==
  In1 : Inport
  R_o_2_i : Inport  Port=2
  W_orbit : Inport  Port=3
  Action Port : ActionPort  ActionPortLabel=case [ 1 ]:
  Out1 : Outport  VectorParamsAs1DForOutWhenUnconnected=off
  Out2 : Outport  Port=2  VectorParamsAs1DForOutWhenUnconnected=off
  Out3 : Outport  Port=3  VectorParamsAs1DForOutWhenUnconnected=off
  wires:
  In1/1 -> Out1/1
  R_o_2_i/1 -> Out2/1
  W_orbit/1 -> Out3/1

== system MEKFsim_v2/Reference/Switch Case Action Subsystem6 ==
  In1 : Inport
  In2 : Inport  Port=2
  Action Port : ActionPort  ActionPortLabel=case [ 7 ]:
  Derivative : Derivative
  Matrix Multiply : Product  Multiplication=Matrix(*)
  Quaternions to Direction Cosine Matrix : sharedtransform/Quaternions to  Direction Cosine Matrix  aMode=aMode
      settings: SourceProductBaseCode=AE,PW,MT,UV,VE,VP
  Transpose : Math  Operator=transpose  SaturateOnIntegerOverflow=on
  Transpose1 : Math  Operator=transpose  SaturateOnIntegerOverflow=on
  gets vector from Skew Matrix : MATLABFcn  MATLABFcn=vec_from_skew
  Out1 : Outport  VectorParamsAs1DForOutWhenUnconnected=off
  Out2 : Outport  Port=2  VectorParamsAs1DForOutWhenUnconnected=off
  W_custom : Outport  Port=3
  wires:
  In1/1 -> Out1/1
  In2/1 -> Quaternions to Direction Cosine Matrix/1
  Quaternions to Direction Cosine Matrix/1 -> Transpose1/1
  Matrix Multiply/1 -> gets vector from Skew Matrix/1
  Transpose/1 -> Derivative/1
  gets vector from Skew Matrix/1 -> W_custom/1
  Derivative/1 -> Matrix Multiply/1
  Transpose1/1 -> Transpose/1, Matrix Multiply/2, Out2/1

== system MEKFsim_v2/Reference/Switch Case Action Subsystem7 ==
  In1 : Inport
  Input1 : Inport  Port=2
  In2 : Inport  Port=3
  Action Port : ActionPort  ActionPortLabel=case [ 6 ]:
  Out1 : Outport  VectorParamsAs1DForOutWhenUnconnected=off
  Out3 : Outport  Port=2  VectorParamsAs1DForOutWhenUnconnected=off
  Out2 : Outport  Port=3  VectorParamsAs1DForOutWhenUnconnected=off
  wires:
  In1/1 -> Out1/1
  Input1/1 -> Out3/1
  In2/1 -> Out2/1

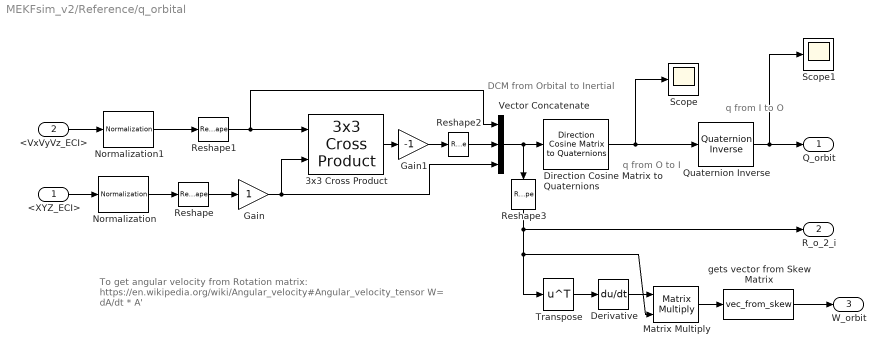
== system MEKFsim_v2/Reference/q_orbital ==
  note: DCM from Orbital to Inertial
  note: q from O to I
  note: q from I to O
  note: To get angular velocity from Rotation matrix:
      | https://en.wikipedia.org/wiki/Angular_velocity#Angular_velocity_tensor
      | W= dA/dt * A'
  <XYZ_ECI> : Inport
  <VxVyVz_ECI> : Inport  Port=2
  3x3 Cross Product : sharedutil/3x3 Cross Product  aMode=aMode
      settings: SourceProductBaseCode=AE,PW,MT,UV,VE,VP
  Derivative : Derivative
  Direction Cosine Matrix to Quaternions : sharedtransform/Direction Cosine Matrix  to Quaternions  aMode=0  action=None  tolerance=eps(2)
      settings: SourceProductBaseCode=AE,PW,MT,UV,VE,VP
  Gain : Gain
  Gain1 : Gain  Gain=-1
  Matrix Multiply : Product  Multiplication=Matrix(*)
  Normalization : dspmathops/Normalization  NormType=2-norm  Bias=1e-10  NormOver=Each column  Dimension=1  roundingMode=Floor  overflowMode=off  accumDataTypeStr=Inherit: Same as product output  accumLastDataTypeStr=Inherit: Same as product output  outputDataTypeStr=Inherit: Same as product output  outputMin=[]  outputMax=[]  outputLastDataTypeStr=Inherit: Same as product output
  Normalization1 : dspmathops/Normalization  NormType=2-norm  Bias=1e-10  NormOver=Each column  Dimension=1  roundingMode=Floor  overflowMode=off  accumDataTypeStr=Inherit: Same as product output  accumLastDataTypeStr=Inherit: Same as product output  outputDataTypeStr=Inherit: Same as product output  outputMin=[]  outputMax=[]  outputLastDataTypeStr=Inherit: Same as product output
  Quaternion Inverse : aerolibutil/Quaternion Inverse
  Reshape : Reshape  OutputDimensionality=Column vector (2-D)
  Reshape1 : Reshape  OutputDimensionality=Column vector (2-D)
  Reshape2 : Reshape  OutputDimensionality=Column vector (2-D)
  Reshape3 : Reshape  OutputDimensionality=Customize  OutputDimensions=[3,3]
  Scope : Scope
  Scope1 : Scope
  Transpose : Math  Operator=transpose  SaturateOnIntegerOverflow=on
  Vector Concatenate : Concatenate  NumInputs=3  Mode=Multidimensional array  ConcatenateDimension=2
  gets vector from Skew Matrix : MATLABFcn  MATLABFcn=vec_from_skew
  Q_orbit : Outport  VectorParamsAs1DForOutWhenUnconnected=off
  R_o_2_i : Outport  Port=2  VectorParamsAs1DForOutWhenUnconnected=off
  W_orbit : Outport  Port=3
  wires:
  Normalization/1 -> Reshape/1
  Normalization1/1 -> Reshape1/1
  <VxVyVz_ECI>/1 -> Normalization1/1
  Reshape1/1 -> 3x3 Cross Product/1, Vector Concatenate/1
  <XYZ_ECI>/1 -> Normalization/1
  Reshape/1 -> Gain/1
  Gain/1 -> 3x3 Cross Product/2, Vector Concatenate/3
  Direction Cosine Matrix to Quaternions/1 -> Scope/1, Quaternion Inverse/1
  3x3 Cross Product/1 -> Gain1/1
  Gain1/1 -> Reshape2/1
  Quaternion Inverse/1 -> Scope1/1, Q_orbit/1
  Vector Concatenate/1 -> Reshape3/1, Direction Cosine Matrix to Quaternions/1
  gets vector from Skew Matrix/1 -> W_orbit/1
  Matrix Multiply/1 -> gets vector from Skew Matrix/1
  Transpose/1 -> Derivative/1
  Derivative/1 -> Matrix Multiply/1
  Reshape2/1 -> Vector Concatenate/2
  Reshape3/1 -> Matrix Multiply/2, Transpose/1, R_o_2_i/1

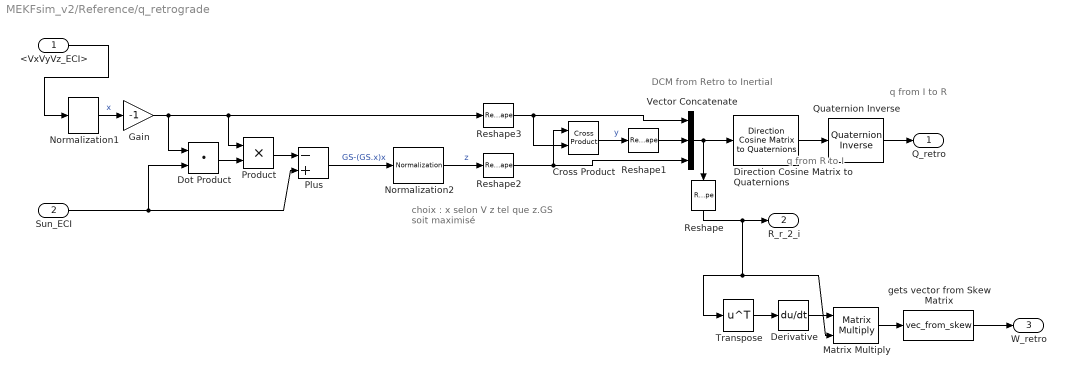
== system MEKFsim_v2/Reference/q_retrograde ==
  note: q from I to R
  note: q from R to I
  note: DCM from Retro to Inertial
  note: choix :
      | x selon V
      | z tel que z.GS soit maximisé
  <VxVyVz_ECI> : Inport
  Sun_ECI : Inport  Port=2
  Cross Product : vrlib/Utilities/Cross Product
  Derivative : Derivative
  Direction Cosine Matrix to Quaternions : sharedtransform/Direction Cosine Matrix  to Quaternions  aMode=0  action=None  tolerance=eps(2)
      settings: SourceProductBaseCode=AE,PW,MT,UV,VE,VP
  Dot Product : DotProduct  InputSameDT=on  OutDataTypeStr=Inherit: Inherit via internal rule
  Gain : Gain  Gain=-1
  Matrix Multiply : Product  Multiplication=Matrix(*)
  Normalization1 : dspmathops/Normalization  NormType=2-norm  Bias=1e-10  NormOver=Each column  Dimension=1  roundingMode=Floor  overflowMode=off  accumDataTypeStr=Inherit: Same as product output  accumLastDataTypeStr=Inherit: Same as product output  outputDataTypeStr=Inherit: Same as product output  outputMin=[]  outputMax=[]  outputLastDataTypeStr=Inherit: Same as product output
  Normalization2 : dspmathops/Normalization  NormType=2-norm  Bias=1e-10  NormOver=Each column  Dimension=1  roundingMode=Floor  overflowMode=off  accumDataTypeStr=Inherit: Same as product output  accumLastDataTypeStr=Inherit: Same as product output  outputDataTypeStr=Inherit: Same as product output  outputMin=[]  outputMax=[]  outputLastDataTypeStr=Inherit: Same as product output
  Plus : Sum  Inputs=-+
  Product : Product
  Quaternion Inverse : aerolibutil/Quaternion Inverse
  Reshape : Reshape  OutputDimensionality=Customize  OutputDimensions=[3,3]
  Reshape1 : Reshape  OutputDimensionality=Column vector (2-D)
  Reshape2 : Reshape  OutputDimensionality=Column vector (2-D)
  Reshape3 : Reshape  OutputDimensionality=Column vector (2-D)
  Transpose : Math  Operator=transpose  SaturateOnIntegerOverflow=on
  Vector Concatenate : Concatenate  NumInputs=3  Mode=Multidimensional array  ConcatenateDimension=2
  gets vector from Skew Matrix : MATLABFcn  MATLABFcn=vec_from_skew
  Q_retro : Outport  VectorParamsAs1DForOutWhenUnconnected=off
  R_r_2_i : Outport  Port=2  VectorParamsAs1DForOutWhenUnconnected=off
  W_retro : Outport  Port=3
  wires:
  Quaternion Inverse/1 -> Q_retro/1
  Reshape2/1 -> Vector Concatenate/3, Cross Product/1
  Reshape3/1 -> Vector Concatenate/1, Cross Product/2
  Product/1 -> Plus/1
  Dot Product/1 -> Product/2
  Cross Product/1 -> Reshape1/1  "y"
  Normalization2/1 -> Reshape2/1  "z"
  Plus/1 -> Normalization2/1  "GS-(GS.x)x"
  Sun_ECI/1 -> Dot Product/2, Plus/2
  Direction Cosine Matrix to Quaternions/1 -> Quaternion Inverse/1
  Normalization1/1 -> Gain/1  "x"
  <VxVyVz_ECI>/1 -> Normalization1/1
  Reshape1/1 -> Vector Concatenate/2
  Gain/1 -> Dot Product/1, Product/1, Reshape3/1
  Vector Concatenate/1 -> Direction Cosine Matrix to Quaternions/1, Reshape/1
  gets vector from Skew Matrix/1 -> W_retro/1
  Matrix Multiply/1 -> gets vector from Skew Matrix/1
  Derivative/1 -> Matrix Multiply/1
  Transpose/1 -> Derivative/1
  Reshape/1 -> Transpose/1, Matrix Multiply/2, R_r_2_i/1

== system MEKFsim_v2/Reference/q_rotation_y_pi//2 ==
  z_ECI : Inport
  V_ECI : Inport  Port=2
  Cross Product : vrlib/Utilities/Cross Product
  Product : Product
  Reshape1 : Reshape  OutputDimensionality=Column vector (2-D)
  Vector Concatenate1 : Concatenate  Mode=Multidimensional array
  cos pi/4 : Constant  Value=[sqrt(2)]
  sin pi/4 : Constant  Value=sqrt(2)
  Q_rot_drag : Outport  VectorParamsAs1DForOutWhenUnconnected=off
  wires:
  cos pi/4/1 -> Vector Concatenate1/1
  Vector Concatenate1/1 -> Q_rot_drag/1
  sin pi/4/1 -> Product/2
  z_ECI/1 -> Cross Product/1
  V_ECI/1 -> Cross Product/2
  Cross Product/1 -> Product/1  "y"
  Reshape1/1 -> Vector Concatenate1/2
  Product/1 -> Reshape1/1

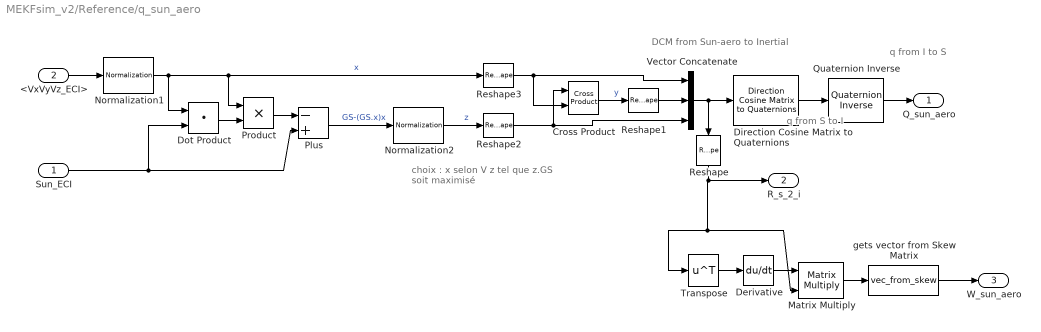
== system MEKFsim_v2/Reference/q_sun_aero ==
  note: q from I to S
  note: q from S to I
  note: DCM from Sun-aero to Inertial
  note: choix :
      | x selon V
      | z tel que z.GS soit maximisé
  Sun_ECI : Inport
  <VxVyVz_ECI> : Inport  Port=2
  Cross Product : vrlib/Utilities/Cross Product
  Derivative : Derivative
  Direction Cosine Matrix to Quaternions : sharedtransform/Direction Cosine Matrix  to Quaternions  aMode=0  action=None  tolerance=eps(2)
      settings: SourceProductBaseCode=AE,PW,MT,UV,VE,VP
  Dot Product : DotProduct  InputSameDT=on  OutDataTypeStr=Inherit: Inherit via internal rule
  Matrix Multiply : Product  Multiplication=Matrix(*)
  Normalization1 : dspmathops/Normalization  NormType=2-norm  Bias=1e-10  NormOver=Each column  Dimension=1  roundingMode=Floor  overflowMode=off  accumDataTypeStr=Inherit: Same as product output  accumLastDataTypeStr=Inherit: Same as product output  outputDataTypeStr=Inherit: Same as product output  outputMin=[]  outputMax=[]  outputLastDataTypeStr=Inherit: Same as product output
  Normalization2 : dspmathops/Normalization  NormType=2-norm  Bias=1e-10  NormOver=Each column  Dimension=1  roundingMode=Floor  overflowMode=off  accumDataTypeStr=Inherit: Same as product output  accumLastDataTypeStr=Inherit: Same as product output  outputDataTypeStr=Inherit: Same as product output  outputMin=[]  outputMax=[]  outputLastDataTypeStr=Inherit: Same as product output
  Plus : Sum  Inputs=-+
  Product : Product
  Quaternion Inverse : aerolibutil/Quaternion Inverse
  Reshape : Reshape  OutputDimensionality=Customize  OutputDimensions=[3,3]
  Reshape1 : Reshape  OutputDimensionality=Column vector (2-D)
  Reshape2 : Reshape  OutputDimensionality=Column vector (2-D)
  Reshape3 : Reshape  OutputDimensionality=Column vector (2-D)
  Transpose : Math  Operator=transpose  SaturateOnIntegerOverflow=on
  Vector Concatenate : Concatenate  NumInputs=3  Mode=Multidimensional array  ConcatenateDimension=2
  gets vector from Skew Matrix : MATLABFcn  MATLABFcn=vec_from_skew
  Q_sun_aero : Outport  VectorParamsAs1DForOutWhenUnconnected=off
  R_s_2_i : Outport  Port=2  VectorParamsAs1DForOutWhenUnconnected=off
  W_sun_aero : Outport  Port=3
  wires:
  Quaternion Inverse/1 -> Q_sun_aero/1
  Reshape2/1 -> Vector Concatenate/3, Cross Product/1
  Reshape3/1 -> Vector Concatenate/1, Cross Product/2
  Product/1 -> Plus/1
  Dot Product/1 -> Product/2
  Cross Product/1 -> Reshape1/1  "y"
  Normalization2/1 -> Reshape2/1  "z"
  Plus/1 -> Normalization2/1  "GS-(GS.x)x"
  Sun_ECI/1 -> Dot Product/2, Plus/2
  Direction Cosine Matrix to Quaternions/1 -> Quaternion Inverse/1
  Normalization1/1 -> Dot Product/1, Product/1, Reshape3/1  "x"
  <VxVyVz_ECI>/1 -> Normalization1/1
  Reshape1/1 -> Vector Concatenate/2
  Transpose/1 -> Derivative/1
  Matrix Multiply/1 -> gets vector from Skew Matrix/1
  Derivative/1 -> Matrix Multiply/1
  Vector Concatenate/1 -> Direction Cosine Matrix to Quaternions/1, Reshape/1
  gets vector from Skew Matrix/1 -> W_sun_aero/1
  Reshape/1 -> Transpose/1, Matrix Multiply/2, R_s_2_i/1

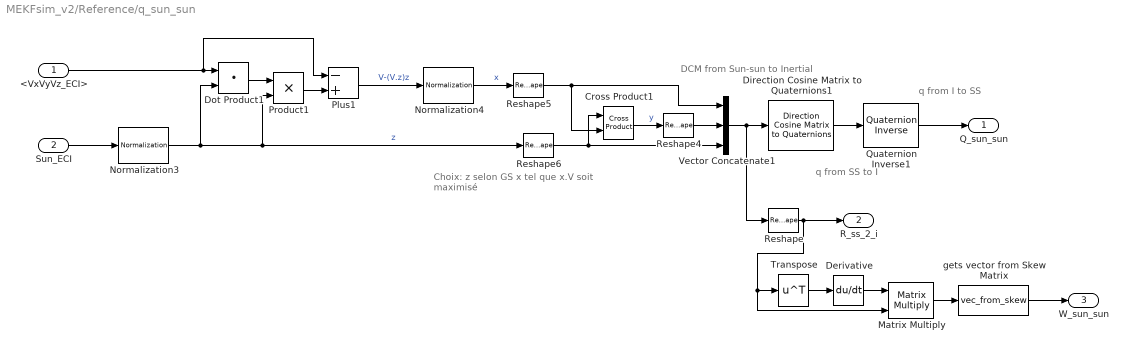
== system MEKFsim_v2/Reference/q_sun_sun ==
  note: Choix:
      | z selon GS
      | x tel que x.V soit maximisé
  note: DCM from Sun-sun to Inertial
  note: q from I to SS
  note: q from SS to I
  <VxVyVz_ECI> : Inport
  Sun_ECI : Inport  Port=2
  Cross Product1 : vrlib/Utilities/Cross Product
  Derivative : Derivative
  Direction Cosine Matrix to Quaternions1 : sharedtransform/Direction Cosine Matrix  to Quaternions  aMode=0  action=None  tolerance=eps(2)
      settings: SourceProductBaseCode=AE,PW,MT,UV,VE,VP
  Dot Product1 : DotProduct  InputSameDT=on  OutDataTypeStr=Inherit: Inherit via internal rule
  Matrix Multiply : Product  Multiplication=Matrix(*)
  Normalization3 : dspmathops/Normalization  NormType=2-norm  Bias=1e-10  NormOver=Each column  Dimension=1  roundingMode=Floor  overflowMode=off  accumDataTypeStr=Inherit: Same as product output  accumLastDataTypeStr=Inherit: Same as product output  outputDataTypeStr=Inherit: Same as product output  outputMin=[]  outputMax=[]  outputLastDataTypeStr=Inherit: Same as product output
  Normalization4 : dspmathops/Normalization  NormType=2-norm  Bias=1e-10  NormOver=Each column  Dimension=1  roundingMode=Floor  overflowMode=off  accumDataTypeStr=Inherit: Same as product output  accumLastDataTypeStr=Inherit: Same as product output  outputDataTypeStr=Inherit: Same as product output  outputMin=[]  outputMax=[]  outputLastDataTypeStr=Inherit: Same as product output
  Plus1 : Sum  Inputs=-+
  Product1 : Product
  Quaternion Inverse1 : aerolibutil/Quaternion Inverse
  Reshape : Reshape  OutputDimensionality=Customize  OutputDimensions=[3,3]
  Reshape4 : Reshape  OutputDimensionality=Column vector (2-D)
  Reshape5 : Reshape  OutputDimensionality=Column vector (2-D)
  Reshape6 : Reshape  OutputDimensionality=Column vector (2-D)
  Transpose : Math  Operator=transpose  SaturateOnIntegerOverflow=on
  Vector Concatenate1 : Concatenate  NumInputs=3  Mode=Multidimensional array  ConcatenateDimension=2
  gets vector from Skew Matrix : MATLABFcn  MATLABFcn=vec_from_skew
  Q_sun_sun : Outport  VectorParamsAs1DForOutWhenUnconnected=off
  R_ss_2_i : Outport  Port=2  VectorParamsAs1DForOutWhenUnconnected=off
  W_sun_sun : Outport  Port=3
  wires:
  Direction Cosine Matrix to Quaternions1/1 -> Quaternion Inverse1/1
  Reshape4/1 -> Vector Concatenate1/2
  Dot Product1/1 -> Product1/1
  Sun_ECI/1 -> Normalization3/1
  Quaternion Inverse1/1 -> Q_sun_sun/1
  <VxVyVz_ECI>/1 -> Dot Product1/1, Plus1/1
  Plus1/1 -> Normalization4/1  "V-(V.z)z"
  Reshape6/1 -> Cross Product1/1, Vector Concatenate1/3
  Normalization3/1 -> Dot Product1/2, Product1/2, Reshape6/1  "z"
  Reshape5/1 -> Cross Product1/2, Vector Concatenate1/1
  Cross Product1/1 -> Reshape4/1  "y"
  Normalization4/1 -> Reshape5/1  "x"
  Product1/1 -> Plus1/2
  Reshape/1 -> Matrix Multiply/2, Transpose/1, R_ss_2_i/1
  Derivative/1 -> Matrix Multiply/1
  Transpose/1 -> Derivative/1
  Matrix Multiply/1 -> gets vector from Skew Matrix/1
  gets vector from Skew Matrix/1 -> W_sun_sun/1
  Vector Concatenate1/1 -> Direction Cosine Matrix to Quaternions1/1, Reshape/1
